simulink model "Realtime_udp_module"  (R2016a)
settings: Solver=ode3  StartTime=0.0  StopTime=inf  FixedStep=dt  RelTol=1e-3
InitFcn:
  | PSMCMD_DEPENDENCY
  | init_psm_cmd
  | init_scopes
  | init_udp
  | init_resolved_rates
  | ATI_Init_gamma
undefined symbols (not defined in the file or in its folder): H_organ2robot, H_robot2organ, R_organ2robot, R_robot2organ, Rft2organ
libraries: xpcobsoletelib x2, xpcrtudplib x2, xpciplib x1
settings Model: xpc_rtwmakecfg_data=_xpcetherlib__xpcether8255xlib__xpcetherGbElib_  Creator=Andrea  LastModifiedBy=Long
settings SolverCC: EnableConcurrentExecution=on
settings DataIOCC: LimitDataPoints=on  SaveFormat=Array  SignalLoggingSaveFormat=ModelDataLogs
settings OptimizationCC: BlockReduction=off  OptimizeBlockIOStorage=off  BufferReuse=off  GlobalBufferReuse=off  ExpressionFolding=off  ExpressionDepthLimit=2147483647  LocalBlockOutputs=off  OptimizeModelRefInitCode=on
settings DebuggingCC: UnderspecifiedInitializationDetection=Classic  MergeDetectMultiDrivingBlocksExec=none  SolverPrmCheckMsg=warning  MultiTaskCondExecSysMsg=warning  MultiTaskRateTransMsg=warning  FcnCallInpInsideContextMsg=UseLocalSettings  StateNameClashWarn=warning
settings HardwareCC: ProdBitPerPointer=32  ProdLargestAtomicFloat=None  ProdWordSize=32  ProdLongLongMode=on  ProdHWDeviceType=Generic->32-bit x86 compatible
settings ModelReferenceCC: PropagateSignalLabelsOutOfModel=off
settings SFSimCC: SimParseCustomCode=off
settings RTWCC: SystemTargetFile=slrtert.tlc  TemplateMakefile=slrtert_default_tmf  Description=Simulink Real-Time (ERT)  RTWCompilerOptimization=on
settings CodeAppCC: CustomSymbolStrType=$N$R$M  InternalIdentifier=Classic
settings SimulinkRealTimeERTCC: TargetFcnLib=ansi_tfl_table_tmw.mat  GenFloatMathFcnCalls=NOT IN USE  TargetLangStandard=C89/C90 (ANSI)  CodeReplacementLibrary=XPC_BLAS  UtilityFuncGeneration=Auto  ERTMultiwordTypeDef=System defined  ERTMultiwordLength=256  MultiwordLength=2048  GenerateFullHeader=on  InferredTypesCompatibility=off  GenerateSampleERTMain=off  GenerateTestInterfaces=off  ModelReferenceCompliant=on  ParMdlRefBuildCompliant=on  CompOptLevelCompliant=on  ConcurrentExecutionCompliant=on  IncludeMdlTerminateFcn=on  GeneratePreprocessorConditionals=Disable all  CombineOutputUpdateFcns=off  CombineSignalStateStructs=off  SuppressErrorStatus=off  ERTFirstTimeCompliant=off  IncludeFileDelimiter=Auto  ERTCustomFileBanners=off  SupportAbsoluteTime=on  LogVarNameModifier=rt_  MatFileLogging=on  MultiInstanceERTCode=off  CodeInterfacePackaging=Nonreusable function  SupportNonFinite=on  SupportComplex=on  PurelyIntegerCode=off  SupportContinuousTime=on  SupportNonInlinedSFcns=on  SupportVariableSizeSignals=off  ParenthesesLevel=Nominal  CastingMode=Nominal  MATLABClassNameForMDSCustomization=xpcAperiodicCustomization  ModelStepFunctionPrototypeControlCompliant=off  CPPClassGenCompliant=off  AutosarCompliant=off  GRTInterface=on  GenerateAllocFcn=off  UseToolchainInfoCompliant=off  GenerateSharedConstants=on  ExtModeTransport=0  ExtModeStaticAlloc=off  ExtModeStaticAllocSize=1000000  ExtModeTesting=off  InlinedParameterPlacement=Hierarchical  TargetOS=BareBoardExample  MultiInstanceErrorCode=Error  RateGroupingCode=on  RootIOFormat=Individual arguments  RTWCAPIRootIO=off  EnableDataOwnership=off  ERTFilePackagingFormat=Modular  PreserveExpressionOrder=off  PreserveIfCondition=off  ConvertIfToSwitch=off  PreserveExternInFcnDecls=on  SuppressUnreachableDefaultCases=off  EnableSignedLeftShifts=on  EnableSignedRightShifts=on  IndentStyle=K&R  IndentSize=2  EnableUserReplacementTypes=off  MaxIdInt32=MAX_int32_T  MinIdInt32=MIN_int32_T  MaxIdUint32=MAX_uint32_T  MaxIdInt16=MAX_int16_T  MinIdInt16=MIN_int16_T  MaxIdUint16=MAX_uint16_T  MaxIdInt8=MAX_int8_T  MinIdInt8=MIN_int8_T  MaxIdUint8=MAX_uint8_T  BooleanTrueId=true  BooleanFalseId=false  MemSecPackage=--- None ---  MemSecDataConstants=Default  MemSecDataIO=Default  MemSecDataInternal=Default  MemSecDataParameters=Default  MemSecFuncInitTerm=Default  MemSecFuncExecute=Default  MemSecFuncSharedUtil=Default  GlobalDataDefinition=Auto  GlobalDataReference=Auto  GenerateASAP2=off  ERTSrcFileBannerTemplate=ert_code_template.cgt  ERTHdrFileBannerTemplate=ert_code_template.cgt  ERTDataSrcFileTemplate=ert_code_template.cgt  ERTDataHdrFileTemplate=ert_code_template.cgt  ERTCustomFileTemplate=example_file_process.tlc  SignalDisplayLevel=10  ParamTuneLevel=10  InitialValueSource=Model  RTWCAPISignals=off  RTWCAPIParams=on  RTWCAPIStates=off  RL32ModeModifier=Real-Time  ExtMode=on  ExtModeMexFile=ext_xpc  ExtModeIntrfLevel=Level2 - Open  ExtModeArmWhenConnect=off  RL32LogTETModifier=on  RL32LogBufSizeModifier=100000  xPCTaskExecutionProfile=off  xPCRL32EventNumber=5000  RL32IRQSourceModifier=Timer  xPCIRQSourceBoard=None/Other  xPCIOIRQSlot=-1  xpcObjCom=off  xPCGenerateASAP2=off  xPCGenerateXML=off  RL32ObjectName=tg  xPCisDownloadable=off  xPCisDefaultEnv=on  xPCisModelTimeout=on  xPCModelTimeoutSecs=5  xpcDblBuff=off  xPCLoadParamSetFile=off  xPCConcurrentTasks=off  xPCEnableSFAnimation=off
settings ConfigComp: CovModelRefEnable=Off

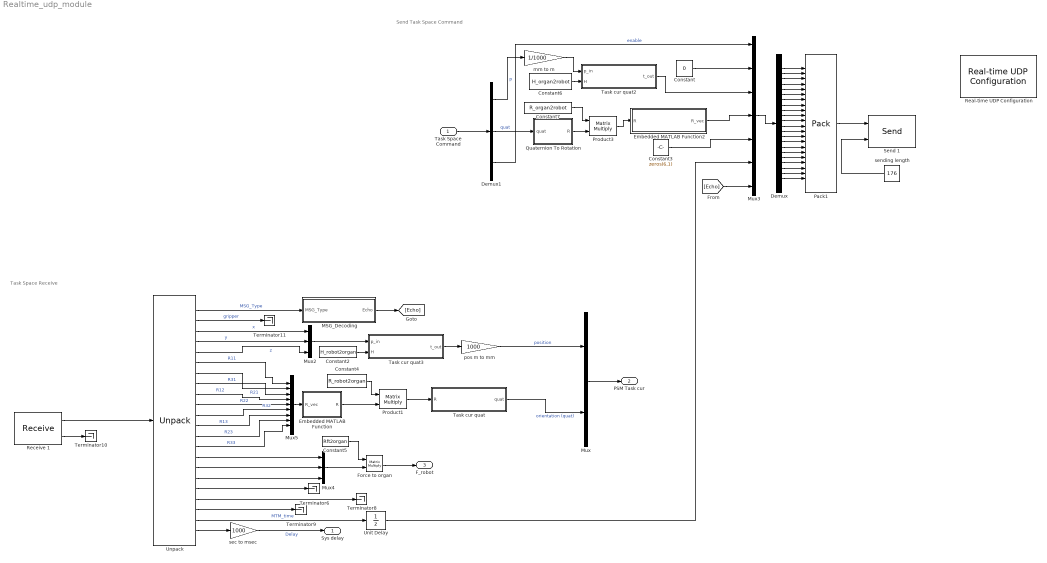
== system Realtime_udp_module ==
  note: Task Space Receive
  note: Send Task Space Command
  Task Space Command : Inport
  Constant : Constant  Value=0
  Constant2 : Constant  Value=H_robot2organ
  Constant3 : Constant  Value=zeros(6,1)
  Constant4 : Constant  Value=R_robot2organ
  Constant5 : Constant  Value=Rft2organ
  Constant6 : Constant  Value=H_organ2robot
  Constant7 : Constant  Value=R_organ2robot
  Demux : Demux  Outputs=22
  Demux1 : Demux  Outputs=[3,4,1]
  Embedded MATLAB Function : MATLAB Function  TreatAsAtomicUnit=on
  Embedded MATLAB Function2 : MATLAB Function  TreatAsAtomicUnit=on
  Force to organ : Product  Multiplication=Matrix(*)
  MSG_Decoding : MATLAB Function  TreatAsAtomicUnit=on
  Mux : Mux  Inputs=[3,4]
  Mux2 : Mux  Inputs=3
  Mux3 : Mux  Inputs=7
  Mux4 : Mux  Inputs=3
  Mux5 : Mux  Inputs=9
  Pack1 : xpcobsoletelib/Utilities/Pack   datatypes={'double' 'double' 'double' 'double' 'double' 'double' 'double' 'double' 'double' 'double' 'double' 'double' 'double' 'double' 'double' 'double' 'double' 'double' 'double' 'double' 'double' 'double'}  byteAlign=1
  Product1 : Product  Multiplication=Matrix(*)
  Product3 : Product  Multiplication=Matrix(*)
  Quaternion To Rotation : MATLAB Function  TreatAsAtomicUnit=on
  "Real-time UDP Configuration " : xpciplib/Real-time UDP  Configuration   ID=2  IpAddress=191.167.2.202  SubnetMask=255.255.255.0  Gateway=255.255.255.255  EthDrv=Intel Gigabit  PciBus=5  PciSlot=0  udpID=0  MulticastList=[]  Multicast={}
  Receive 1 : xpcrtudplib/Receive   ID=2  Receive1=0.0.0.0  Receive2=10006  Receive3=22*8  Receive4=dt_udp  udpID=0
  Send 1 : xpcrtudplib/Send   ID=2  Send1=192.168.1.11  Send2=10005  Send3=-1  Send4=dt_udp  udpID=0
  Task cur quat : MATLAB Function  TreatAsAtomicUnit=on
  Task cur quat2 : MATLAB Function  TreatAsAtomicUnit=on
  Task cur quat3 : MATLAB Function  TreatAsAtomicUnit=on
  Terminator{6,8..11} (5 alike) : Terminator
  Unit Delay : UnitDelay  SampleTime=-1
  Unpack : xpcobsoletelib/Utilities/Unpack   dimensions={1,1,1,1,1,1,1,1,1,1,1,1,1,1,1,1,1,1,1,1,1,1}  datatypes={'double' 'double' 'double' 'double' 'double' 'double' 'double' 'double' 'double' 'double' 'double' 'double' 'double' 'double' 'double' 'double' 'double' 'double' 'double' 'double' 'double' 'double'}  byteAlign=1
  mm to m : Gain  Gain=1/1000
  pos m to mm : Gain  Gain=1000
  sec to msec : Gain  Gain=1000
  sending length : Constant  Value=176
  Sys delay : Outport
  PSM Task cur : Outport  Port=2
  F_robot : Outport  Port=3
  wires:
  Task Space Command/1 -> Demux1/1
  Mux/1 -> PSM Task cur/1
  Unpack/19 -> Terminator8/1
  Unpack/20 -> Terminator9/1
  Unpack/18 -> Terminator6/1
  Unpack/17 -> Mux4/3
  Unpack/16 -> Mux4/2
  Unpack/15 -> Mux4/1
  Mux5/1 -> Embedded MATLAB Function/1(R_vec)
  Unpack/14 -> Mux5/9  "R33"
  Unpack/13 -> Mux5/8  "R23"
  Unpack/12 -> Mux5/7  "R13"
  Unpack/11 -> Mux5/6  "R32"
  Unpack/10 -> Mux5/5  "R22"
  Unpack/9 -> Mux5/4  "R12"
  Unpack/8 -> Mux5/3  "R31"
  Unpack/7 -> Mux5/2  "R21"
  Unpack/6 -> Mux5/1  "R11"
  Unpack/22 -> sec to msec/1
  Mux2/1 -> Task cur quat3/1(p_in)
  Unpack/3 -> Mux2/1  "x"
  Unpack/4 -> Mux2/2  "y"
  Unpack/5 -> Mux2/3  "z"
  Receive 1/1 -> Unpack/1
  Unpack/1 -> MSG_Decoding/1(MSG_Type)  "MSG_Type"
  Unpack/2 -> Terminator11/1  "gripper"
  pos m to mm/1 -> Mux/1  "position"
  Unpack/21 -> Unit Delay/1  "MTM_time"
  Receive 1/2 -> Terminator10/1
  Task cur quat/1(quat) -> Mux/2  "orientation (quat)"
  Pack1/1 -> Send 1/1
  Mux3/1 -> Demux/1
  Demux/1 -> Pack1/1
  Demux/2 -> Pack1/2
  Demux/3 -> Pack1/3
  Demux/4 -> Pack1/4
  Demux/5 -> Pack1/5
  Demux/6 -> Pack1/6
  Demux/7 -> Pack1/7
  Demux/8 -> Pack1/8
  Demux/9 -> Pack1/9
  Demux/10 -> Pack1/10
  Demux/11 -> Pack1/11
  Demux/12 -> Pack1/12
  Demux/13 -> Pack1/13
  Demux/14 -> Pack1/14
  Demux/15 -> Pack1/15
  Demux/16 -> Pack1/16
  Demux/17 -> Pack1/17
  Demux/18 -> Pack1/18
  Demux/19 -> Pack1/19
  Demux/20 -> Pack1/20
  Demux/21 -> Pack1/21
  Demux1/2 -> Quaternion To Rotation/1(quat)  "quat"
  Quaternion To Rotation/1(R) -> Product3/2
  MSG_Decoding/1(Echo) -> [Echo]
  [Echo] -> Mux3/7
  Constant/1 -> Mux3/2
  Demux1/1 -> mm to m/1  "p"
  Embedded MATLAB Function2/1(R_vec) -> Mux3/4
  Unit Delay/1 -> Mux3/6
  Constant3/1 -> Mux3/5
  Task cur quat2/1(t_out) -> Mux3/3
  sec to msec/1 -> Sys delay/1  "Delay"
  Demux1/3 -> Mux3/1  "enable"
  Demux/22 -> Pack1/22
  Mux4/1 -> Force to organ/2
  mm to m/1 -> Task cur quat2/1(p_in)
  Constant2/1 -> Task cur quat3/2(H)
  Constant4/1 -> Product1/1
  Embedded MATLAB Function/1(R) -> Product1/2
  Constant5/1 -> Force to organ/1
  Force to organ/1 -> F_robot/1
  Product3/1 -> Embedded MATLAB Function2/1(R)
  Constant6/1 -> Task cur quat2/2(H)
  Constant7/1 -> Product3/1
  Task cur quat3/1(t_out) -> pos m to mm/1
  Product1/1 -> Task cur quat/1(R)
  sending length/1 -> Send 1/2

== matlab function Realtime_udp_module/Task cur quat2 ==
  data: p_in input; t_out output; H input
function t_out   = pos_Transform(p_in,H)
   t_full = H*[p_in;1];
   t_out=t_full(1:3);
end

== matlab function Realtime_udp_module/Task cur quat3 ==
  data: p_in input; t_out output; H input
function t_out   = pos_Transform(p_in,H)
   t_full = H*[p_in;1];
   t_out=t_full(1:3);
end

== matlab function Realtime_udp_module/MSG_Decoding ==
  data: MSG_Type input; Echo output
function Echo = Decode(MSG_Type)
%#codegen
% decode the message_type
% MSG_Type def
% bit0 = valid massage or not(enable or not)
% bit1 = time stamping requested or not (if should send back the local time or not)
enable = bitand(uint8(floor(MSG_Type)),2);
Echo= double(enable);

== matlab function Realtime_udp_module/Quaternion To Rotation ==
  data: quat input; R output
function R = fcn(quat)
%#eml
if norm(quat)==0
    quat = [1;0;0;0];
end
R = quat2rot(quat);

== matlab function Realtime_udp_module/Embedded MATLAB Function2 ==
  data: R input; R_vec output
function R_vec = R_to_vec(R)
%#eml
%%  This func will cast a [3x3] rotation matrix to [9x1]
%%  The mapping will be column matrix, see for yourself.
R_vec = R(:);

== matlab function Realtime_udp_module/Embedded MATLAB Function ==
  data: R_vec input; R output
function R = parse_rot(R_vec)
%#codegen
if norm(R_vec)==0
    R = eye(3);
else
    R = reshape(R_vec,3,3);
end

== matlab function Realtime_udp_module/Task cur quat ==
  data: R input; quat output
function quat   = convert_rot_to_quat(R)
   quat = rot2quat(R);
end
